simulink model "Quadcopter_CTC"  (R2021a)
settings: Solver=ode4  StartTime=0.0  StopTime=40  FixedStep=0.001  RelTol=1e-5
values from neighbouring files (symbols this model uses):
  IQ_x = 7.5e-3    (= 0.0075)    [Parameters.m]
  IQ_y = 7.5e-3    (= 0.0075)    [Parameters.m]
  IQ_z = 1.3e-2    (= 0.013)    [Parameters.m]
  mQ = 0.650    (= 0.65)    [Parameters.m]
libraries: pid_lib x4
settings Model: Creator=Mohamed Eid  LastModifiedBy=Mohamed Eid
settings DebuggingCC: SignalInfNanChecking=error

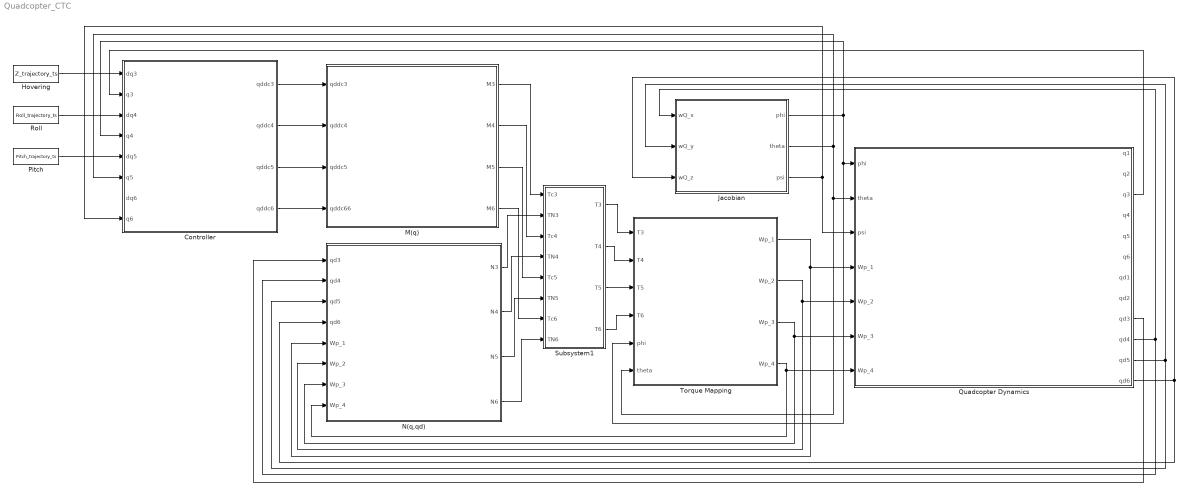
== system Quadcopter_CTC ==
  Controller : Subsystem
  Hovering : FromWorkspace  VariableName=Z_trajectory_ts  SampleTime=-1
  Jacobian : Subsystem
  M(q) : Subsystem
  N(q,qd) : Subsystem
      settings: MinAlgLoopOccurrences=on
  Pitch : FromWorkspace  VariableName=Pitch_trajectory_ts  SampleTime=-1
  Quadcopter Dynamics : Subsystem
      mask Display: image('C:\Users\Mohamed Eid\Desktop\Quadcopter Research\WhatsApp Image 2024-09-17 at 19.38.20.jpeg'); % Use "Edit Image" on toolstrip to change.
  Roll : FromWorkspace  VariableName=Roll_trajectory_ts  SampleTime=-1
  Subsystem1 : Subsystem
      settings: MinAlgLoopOccurrences=on
  Torque Mapping : Subsystem
      settings: MinAlgLoopOccurrences=on
  wires:
  Torque Mapping/3(Wp_3) -> N(q,qd)/7(Wp_3), Quadcopter Dynamics/6(Wp_3)
  Torque Mapping/2(Wp_2) -> N(q,qd)/6(Wp_2), Quadcopter Dynamics/5(Wp_2)
  Torque Mapping/1(Wp_1) -> N(q,qd)/5(Wp_1), Quadcopter Dynamics/4(Wp_1)
  Torque Mapping/4(Wp_4) -> N(q,qd)/8(Wp_4), Quadcopter Dynamics/7(Wp_4)
  Jacobian/1(phi) -> Torque Mapping/5(phi), Quadcopter Dynamics/1(phi), Controller/4(q4)
  Jacobian/2(theta) -> Torque Mapping/6(theta), Quadcopter Dynamics/2(theta), Controller/6(q5)
  Jacobian/3(psi) -> Quadcopter Dynamics/3(psi), Controller/8(q6)
  Quadcopter Dynamics/10(qd4) -> N(q,qd)/2(qd4), Jacobian/1(wQ_x)
  Quadcopter Dynamics/11(qd5) -> N(q,qd)/3(qd5), Jacobian/2(wQ_y)
  Quadcopter Dynamics/12(qd6) -> N(q,qd)/4(qd6), Jacobian/3(wQ_z)
  Controller/1(qddc3) -> M(q)/1(qddc3)
  Controller/2(qddc4) -> M(q)/2(qddc4)
  Controller/3(qddc5) -> M(q)/3(qddc5)
  Controller/4(qddc6) -> M(q)/4(qddc66)
  Quadcopter Dynamics/3(q3) -> Controller/2(q3)
  Quadcopter Dynamics/9(qd3) -> N(q,qd)/1(qd3)
  Subsystem1/1(T3) -> Torque Mapping/1(T3)
  Subsystem1/2(T4) -> Torque Mapping/2(T4)
  Subsystem1/3(T5) -> Torque Mapping/3(T5)
  Subsystem1/4(T6) -> Torque Mapping/4(T6)
  M(q)/1(M3) -> Subsystem1/1(Tc3)
  M(q)/2(M4) -> Subsystem1/3(Tc4)
  M(q)/3(M5) -> Subsystem1/5(Tc5)
  M(q)/4(M6) -> Subsystem1/7(Tc6)
  N(q,qd)/1(N3) -> Subsystem1/2(TN3)
  N(q,qd)/2(N4) -> Subsystem1/4(TN4)
  N(q,qd)/3(N5) -> Subsystem1/6(TN5)
  N(q,qd)/4(N6) -> Subsystem1/8(TN6)
  Hovering/1 -> Controller/1(dq3)
  Roll/1 -> Controller/3(dq4)
  Pitch/1 -> Controller/5(dq5)

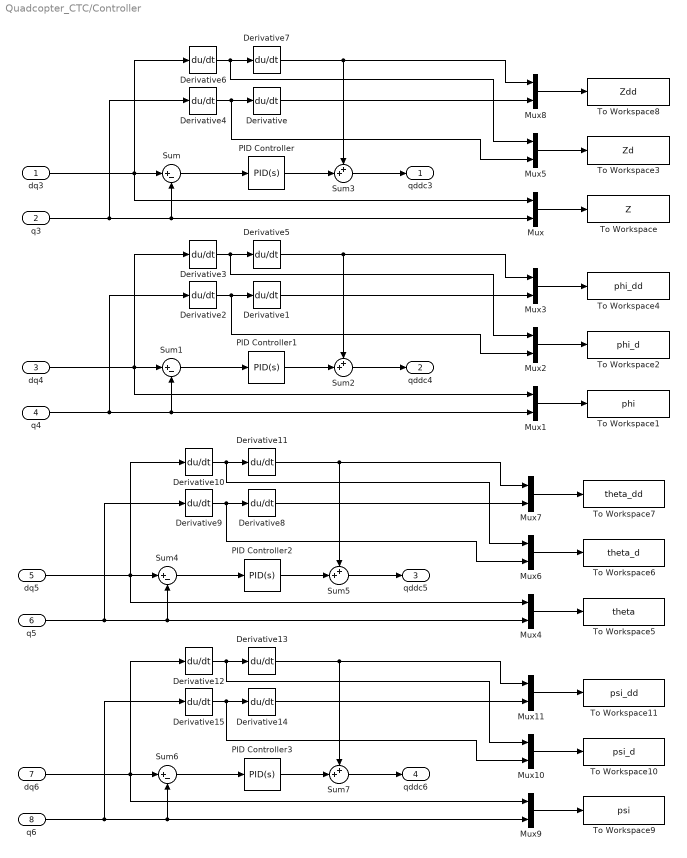
== system Quadcopter_CTC/Controller ==
  dq3 : Inport
  q3 : Inport  Port=2
  dq4 : Inport  Port=3
  q4 : Inport  Port=4
  dq5 : Inport  Port=5
  q5 : Inport  Port=6
  dq6 : Inport  Port=7
  q6 : Inport  Port=8
  Derivative{,1..15} (16 alike) : Derivative
  Mux{,1..11} (12 alike) : Mux  Inputs=2
  PID Controller : pid_lib/PID Controller  Controller=PID  Form=Parallel  TimeDomain=Continuous-time  UseExternalTs=off  SampleTime=-1  IntegratorMethod=Forward Euler  FilterMethod=Forward Euler  ControllerParametersSource=internal  P=2  I=0.6  D=20  UseFilter=on  N=3  TunerSelectOption=Transfer Function Based (PID Tuner App)  InitialConditionSource=internal  InitialConditionForIntegrator=0  InitialConditionForFilter=0  DifferentiatorICPrevScaledInput=0  ExternalReset=none  TrackingMode=off  Kt=1  LimitOutput=off  SatLimitsSource=internal  UpperSaturationLimit=inf  LowerSaturationLimit=-inf  LinearizeAsGain=on  AntiWindupMode=none  Kb=1  POutMin=[]  POutMax=[]  IOutMin=[]  IOutMax=[]  DOutMin=[]  DOutMax=[]  NOutMin=[]  NOutMax=[]  SumOutMin=[]  SumOutMax=[]  SaturationOutMin=[]  SaturationOutMax=[]  PParamMin=[]  PParamMax=[]  IParamMin=[]  IParamMax=[]  DParamMin=[]  DParamMax=[]  NParamMin=[]  NParamMax=[]  KbParamMin=[]  KbParamMax=[]  KtParamMin=[]  KtParamMax=[]  KbOutMin=[]  KbOutMax=[]  KtOutMin=[]  KtOutMax=[]  IntegratorOutMin=[]  IntegratorOutMax=[]  FilterOutMin=[]  FilterOutMax=[]  SumI1OutMin=[]  SumI1OutMax=[]  SumI2OutMin=[]  SumI2OutMax=[]  SumI3OutMin=[]  SumI3OutMax=[]  SumI4OutMin=[]  SumI4OutMax=[]  SumDOutMin=[]  SumDOutMax=[]  DifferentiatorOutMin=[]  DifferentiatorOutMax=[]  FilterDiffOutCoefMin=[]  FilterDiffOutCoefMax=[]  ReciprocalOutMin=[]  ReciprocalOutMax=[]  SumDenOutMin=[]  SumDenOutMax=[]  SumNumOutMin=[]  SumNumOutMax=[]  DivideOutMin=[]  DivideOutMax=[]  UdiffTsProdOutMin=[]  UdiffTsProdOutMax=[]  NTsProdOutMin=[]  NTsProdOutMax=[]  UintegralTsProdOutMin=[]  UintegralTsProdOutMax=[]  UngainTsProdOutMin=[]  UngainTsProdOutMax=[]  IntegratorContinuousStateAttributes=''  IntegratorStateMustResolveToSignalObject=off  IntegratorRTWStateStorageClass=Auto  FilterContinuousStateAttributes=''  FilterStateMustResolveToSignalObject=off  FilterRTWStateStorageClass=Auto  ParallelPVariant=InternalParameters  IdealPVariant=Disabled  IVariant=InternalParameters  DVariant=InternalParameters  IntegratorVariant=Continuous  SatVariant=Disabled  AWVariant=Passthrough  PCopyVariant=Disabled  TRVariant=Disabled  FdbkBlocksVariant=Forward  IdealPFdbkVariant=Disabled  SatFdbkVariant=Disabled  DerivativeFilterVariant=ContFilter  NVariant=InternalParameters  NCopyVariant=Disabled  FilterICVariant=InternalICsFilter  IntegratorICVariant=InternalICs  ExternalResetVariant=Disabled  TRSumVariant=Passthrough  SumFdbkVariant=Disabled  SumVariant=Sum_PID  TsampFilterVariant=InternalTs  TsampNgainVariant=Passthrough  TsampIntegralVariant=Passthrough  ExternalSaturationOutDataTypeStr=Inherit: Same as second input
  PID Controller1 : pid_lib/PID Controller  Controller=PID  Form=Parallel  TimeDomain=Continuous-time  UseExternalTs=off  SampleTime=-1  IntegratorMethod=Forward Euler  FilterMethod=Forward Euler  ControllerParametersSource=internal  P=2.62466504108734  I=0.153121092160732  D=9.99617214845314  UseFilter=on  N=1142.8279760416  TunerSelectOption=Transfer Function Based (PID Tuner App)  InitialConditionSource=internal  InitialConditionForIntegrator=0  InitialConditionForFilter=0  DifferentiatorICPrevScaledInput=0  ExternalReset=none  TrackingMode=off  Kt=1  LimitOutput=off  SatLimitsSource=internal  UpperSaturationLimit=inf  LowerSaturationLimit=-inf  LinearizeAsGain=on  AntiWindupMode=none  Kb=1  POutMin=[]  POutMax=[]  IOutMin=[]  IOutMax=[]  DOutMin=[]  DOutMax=[]  NOutMin=[]  NOutMax=[]  SumOutMin=[]  SumOutMax=[]  SaturationOutMin=[]  SaturationOutMax=[]  PParamMin=[]  PParamMax=[]  IParamMin=[]  IParamMax=[]  DParamMin=[]  DParamMax=[]  NParamMin=[]  NParamMax=[]  KbParamMin=[]  KbParamMax=[]  KtParamMin=[]  KtParamMax=[]  KbOutMin=[]  KbOutMax=[]  KtOutMin=[]  KtOutMax=[]  IntegratorOutMin=[]  IntegratorOutMax=[]  FilterOutMin=[]  FilterOutMax=[]  SumI1OutMin=[]  SumI1OutMax=[]  SumI2OutMin=[]  SumI2OutMax=[]  SumI3OutMin=[]  SumI3OutMax=[]  SumI4OutMin=[]  SumI4OutMax=[]  SumDOutMin=[]  SumDOutMax=[]  DifferentiatorOutMin=[]  DifferentiatorOutMax=[]  FilterDiffOutCoefMin=[]  FilterDiffOutCoefMax=[]  ReciprocalOutMin=[]  ReciprocalOutMax=[]  SumDenOutMin=[]  SumDenOutMax=[]  SumNumOutMin=[]  SumNumOutMax=[]  DivideOutMin=[]  DivideOutMax=[]  UdiffTsProdOutMin=[]  UdiffTsProdOutMax=[]  NTsProdOutMin=[]  NTsProdOutMax=[]  UintegralTsProdOutMin=[]  UintegralTsProdOutMax=[]  UngainTsProdOutMin=[]  UngainTsProdOutMax=[]  IntegratorContinuousStateAttributes=''  IntegratorStateMustResolveToSignalObject=off  IntegratorRTWStateStorageClass=Auto  FilterContinuousStateAttributes=''  FilterStateMustResolveToSignalObject=off  FilterRTWStateStorageClass=Auto  ParallelPVariant=InternalParameters  IdealPVariant=Disabled  IVariant=InternalParameters  DVariant=InternalParameters  IntegratorVariant=Continuous  SatVariant=Disabled  AWVariant=Passthrough  PCopyVariant=Disabled  TRVariant=Disabled  FdbkBlocksVariant=Forward  IdealPFdbkVariant=Disabled  SatFdbkVariant=Disabled  DerivativeFilterVariant=ContFilter  NVariant=InternalParameters  NCopyVariant=Disabled  FilterICVariant=InternalICsFilter  IntegratorICVariant=InternalICs  ExternalResetVariant=Disabled  TRSumVariant=Passthrough  SumFdbkVariant=Disabled  SumVariant=Sum_PID  TsampFilterVariant=InternalTs  TsampNgainVariant=Passthrough  TsampIntegralVariant=Passthrough  ExternalSaturationOutDataTypeStr=Inherit: Same as second input
  PID Controller2 : pid_lib/PID Controller  Controller=PID  Form=Parallel  TimeDomain=Continuous-time  UseExternalTs=off  SampleTime=-1  IntegratorMethod=Forward Euler  FilterMethod=Forward Euler  ControllerParametersSource=internal  P=2.39372296715018  I=0.133362896126307  D=9.54627029036672  UseFilter=on  N=1091.39224421761  TunerSelectOption=Transfer Function Based (PID Tuner App)  InitialConditionSource=internal  InitialConditionForIntegrator=0  InitialConditionForFilter=0  DifferentiatorICPrevScaledInput=0  ExternalReset=none  TrackingMode=off  Kt=1  LimitOutput=off  SatLimitsSource=internal  UpperSaturationLimit=inf  LowerSaturationLimit=-inf  LinearizeAsGain=on  AntiWindupMode=none  Kb=1  POutMin=[]  POutMax=[]  IOutMin=[]  IOutMax=[]  DOutMin=[]  DOutMax=[]  NOutMin=[]  NOutMax=[]  SumOutMin=[]  SumOutMax=[]  SaturationOutMin=[]  SaturationOutMax=[]  PParamMin=[]  PParamMax=[]  IParamMin=[]  IParamMax=[]  DParamMin=[]  DParamMax=[]  NParamMin=[]  NParamMax=[]  KbParamMin=[]  KbParamMax=[]  KtParamMin=[]  KtParamMax=[]  KbOutMin=[]  KbOutMax=[]  KtOutMin=[]  KtOutMax=[]  IntegratorOutMin=[]  IntegratorOutMax=[]  FilterOutMin=[]  FilterOutMax=[]  SumI1OutMin=[]  SumI1OutMax=[]  SumI2OutMin=[]  SumI2OutMax=[]  SumI3OutMin=[]  SumI3OutMax=[]  SumI4OutMin=[]  SumI4OutMax=[]  SumDOutMin=[]  SumDOutMax=[]  DifferentiatorOutMin=[]  DifferentiatorOutMax=[]  FilterDiffOutCoefMin=[]  FilterDiffOutCoefMax=[]  ReciprocalOutMin=[]  ReciprocalOutMax=[]  SumDenOutMin=[]  SumDenOutMax=[]  SumNumOutMin=[]  SumNumOutMax=[]  DivideOutMin=[]  DivideOutMax=[]  UdiffTsProdOutMin=[]  UdiffTsProdOutMax=[]  NTsProdOutMin=[]  NTsProdOutMax=[]  UintegralTsProdOutMin=[]  UintegralTsProdOutMax=[]  UngainTsProdOutMin=[]  UngainTsProdOutMax=[]  IntegratorContinuousStateAttributes=''  IntegratorStateMustResolveToSignalObject=off  IntegratorRTWStateStorageClass=Auto  FilterContinuousStateAttributes=''  FilterStateMustResolveToSignalObject=off  FilterRTWStateStorageClass=Auto  ParallelPVariant=InternalParameters  IdealPVariant=Disabled  IVariant=InternalParameters  DVariant=InternalParameters  IntegratorVariant=Continuous  SatVariant=Disabled  AWVariant=Passthrough  PCopyVariant=Disabled  TRVariant=Disabled  FdbkBlocksVariant=Forward  IdealPFdbkVariant=Disabled  SatFdbkVariant=Disabled  DerivativeFilterVariant=ContFilter  NVariant=InternalParameters  NCopyVariant=Disabled  FilterICVariant=InternalICsFilter  IntegratorICVariant=InternalICs  ExternalResetVariant=Disabled  TRSumVariant=Passthrough  SumFdbkVariant=Disabled  SumVariant=Sum_PID  TsampFilterVariant=InternalTs  TsampNgainVariant=Passthrough  TsampIntegralVariant=Passthrough  ExternalSaturationOutDataTypeStr=Inherit: Same as second input
  PID Controller3 : pid_lib/PID Controller  Controller=PID  Form=Parallel  TimeDomain=Continuous-time  UseExternalTs=off  SampleTime=-1  IntegratorMethod=Forward Euler  FilterMethod=Forward Euler  ControllerParametersSource=internal  P=2.62466504110809  I=0.153121092161943  D=9.99617214853218  UseFilter=on  N=1142.8279760416  TunerSelectOption=Transfer Function Based (PID Tuner App)  InitialConditionSource=internal  InitialConditionForIntegrator=0  InitialConditionForFilter=0  DifferentiatorICPrevScaledInput=0  ExternalReset=none  TrackingMode=off  Kt=1  LimitOutput=off  SatLimitsSource=internal  UpperSaturationLimit=inf  LowerSaturationLimit=-inf  LinearizeAsGain=on  AntiWindupMode=none  Kb=1  POutMin=[]  POutMax=[]  IOutMin=[]  IOutMax=[]  DOutMin=[]  DOutMax=[]  NOutMin=[]  NOutMax=[]  SumOutMin=[]  SumOutMax=[]  SaturationOutMin=[]  SaturationOutMax=[]  PParamMin=[]  PParamMax=[]  IParamMin=[]  IParamMax=[]  DParamMin=[]  DParamMax=[]  NParamMin=[]  NParamMax=[]  KbParamMin=[]  KbParamMax=[]  KtParamMin=[]  KtParamMax=[]  KbOutMin=[]  KbOutMax=[]  KtOutMin=[]  KtOutMax=[]  IntegratorOutMin=[]  IntegratorOutMax=[]  FilterOutMin=[]  FilterOutMax=[]  SumI1OutMin=[]  SumI1OutMax=[]  SumI2OutMin=[]  SumI2OutMax=[]  SumI3OutMin=[]  SumI3OutMax=[]  SumI4OutMin=[]  SumI4OutMax=[]  SumDOutMin=[]  SumDOutMax=[]  DifferentiatorOutMin=[]  DifferentiatorOutMax=[]  FilterDiffOutCoefMin=[]  FilterDiffOutCoefMax=[]  ReciprocalOutMin=[]  ReciprocalOutMax=[]  SumDenOutMin=[]  SumDenOutMax=[]  SumNumOutMin=[]  SumNumOutMax=[]  DivideOutMin=[]  DivideOutMax=[]  UdiffTsProdOutMin=[]  UdiffTsProdOutMax=[]  NTsProdOutMin=[]  NTsProdOutMax=[]  UintegralTsProdOutMin=[]  UintegralTsProdOutMax=[]  UngainTsProdOutMin=[]  UngainTsProdOutMax=[]  IntegratorContinuousStateAttributes=''  IntegratorStateMustResolveToSignalObject=off  IntegratorRTWStateStorageClass=Auto  FilterContinuousStateAttributes=''  FilterStateMustResolveToSignalObject=off  FilterRTWStateStorageClass=Auto  ParallelPVariant=InternalParameters  IdealPVariant=Disabled  IVariant=InternalParameters  DVariant=InternalParameters  IntegratorVariant=Continuous  SatVariant=Disabled  AWVariant=Passthrough  PCopyVariant=Disabled  TRVariant=Disabled  FdbkBlocksVariant=Forward  IdealPFdbkVariant=Disabled  SatFdbkVariant=Disabled  DerivativeFilterVariant=ContFilter  NVariant=InternalParameters  NCopyVariant=Disabled  FilterICVariant=InternalICsFilter  IntegratorICVariant=InternalICs  ExternalResetVariant=Disabled  TRSumVariant=Passthrough  SumFdbkVariant=Disabled  SumVariant=Sum_PID  TsampFilterVariant=InternalTs  TsampNgainVariant=Passthrough  TsampIntegralVariant=Passthrough  ExternalSaturationOutDataTypeStr=Inherit: Same as second input
  Sum{,1,4,6} (4 alike) : Sum  Inputs=|+-
  Sum{2..3,5,7} (4 alike) : Sum  Inputs=++|
  To Workspace : ToWorkspace  VariableName=Z  SaveFormat=Timeseries  SampleTime=-1
  To Workspace1 : ToWorkspace  VariableName=phi  SaveFormat=Timeseries  SampleTime=-1
  To Workspace10 : ToWorkspace  VariableName=psi_d  SaveFormat=Timeseries  SampleTime=-1
  To Workspace11 : ToWorkspace  VariableName=psi_dd  SaveFormat=Timeseries  SampleTime=-1
  To Workspace2 : ToWorkspace  VariableName=phi_d  SaveFormat=Timeseries  SampleTime=-1
  To Workspace3 : ToWorkspace  VariableName=Zd  SaveFormat=Timeseries  SampleTime=-1
  To Workspace4 : ToWorkspace  VariableName=phi_dd  SaveFormat=Timeseries  SampleTime=-1
  To Workspace5 : ToWorkspace  VariableName=theta  SaveFormat=Timeseries  SampleTime=-1
  To Workspace6 : ToWorkspace  VariableName=theta_d  SaveFormat=Timeseries  SampleTime=-1
  To Workspace7 : ToWorkspace  VariableName=theta_dd  SaveFormat=Timeseries  SampleTime=-1
  To Workspace8 : ToWorkspace  VariableName=Zdd  SaveFormat=Timeseries  SampleTime=-1
  To Workspace9 : ToWorkspace  VariableName=psi  SaveFormat=Timeseries  SampleTime=-1
  qddc3 : Outport
  qddc4 : Outport  Port=2
  qddc5 : Outport  Port=3
  qddc6 : Outport  Port=4
  wires:
  Derivative6/1 -> Mux5/1, Derivative7/1
  q3/1 -> Derivative4/1, Sum/2, Mux/2
  Derivative7/1 -> Sum3/1, Mux8/1
  Mux8/1 -> To Workspace8/1
  Mux/1 -> To Workspace/1
  Mux5/1 -> To Workspace3/1
  Sum3/1 -> qddc3/1
  Derivative/1 -> Mux8/2
  dq3/1 -> Derivative6/1, Mux/1, Sum/1
  Derivative4/1 -> Mux5/2, Derivative/1
  Derivative2/1 -> Derivative1/1, Mux2/2
  dq4/1 -> Sum1/1, Mux1/1, Derivative3/1
  Derivative1/1 -> Mux3/2
  Sum2/1 -> qddc4/1
  Mux2/1 -> To Workspace2/1
  Mux1/1 -> To Workspace1/1
  Mux3/1 -> To Workspace4/1
  Derivative5/1 -> Mux3/1, Sum2/1
  q4/1 -> Mux1/2, Sum1/2, Derivative2/1
  Derivative3/1 -> Derivative5/1, Mux2/1
  Derivative10/1 -> Mux6/1, Derivative11/1
  q5/1 -> Derivative9/1, Sum4/2, Mux4/2
  Derivative11/1 -> Sum5/1, Mux7/1
  Mux7/1 -> To Workspace7/1
  PID Controller2/1 -> Sum5/2
  Mux4/1 -> To Workspace5/1
  Mux6/1 -> To Workspace6/1
  Sum5/1 -> qddc5/1
  Derivative8/1 -> Mux7/2
  dq5/1 -> Derivative10/1, Mux4/1, Sum4/1
  Derivative9/1 -> Mux6/2, Derivative8/1
  Sum4/1 -> PID Controller2/1
  Sum6/1 -> PID Controller3/1
  Derivative15/1 -> Derivative14/1, Mux10/2
  dq6/1 -> Sum6/1, Mux9/1, Derivative12/1
  Derivative14/1 -> Mux11/2
  Sum7/1 -> qddc6/1
  Mux10/1 -> To Workspace10/1
  Mux9/1 -> To Workspace9/1
  PID Controller3/1 -> Sum7/2
  Mux11/1 -> To Workspace11/1
  Derivative13/1 -> Mux11/1, Sum7/1
  q6/1 -> Mux9/2, Sum6/2, Derivative15/1
  Derivative12/1 -> Derivative13/1, Mux10/1
  PID Controller1/1 -> Sum2/2
  Sum1/1 -> PID Controller1/1
  PID Controller/1 -> Sum3/2
  Sum/1 -> PID Controller/1

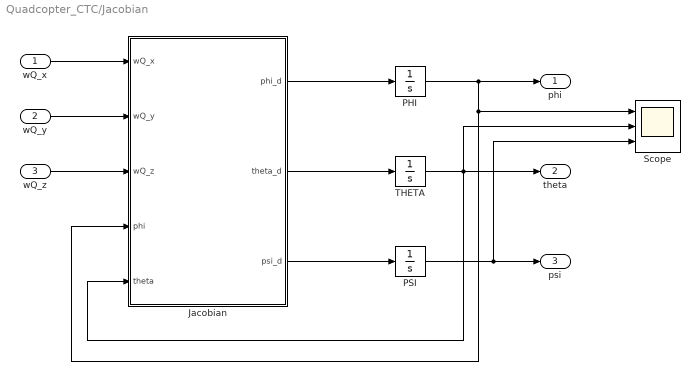
== system Quadcopter_CTC/Jacobian ==
  wQ_x : Inport
  wQ_y : Inport  Port=2
  wQ_z : Inport  Port=3
  Jacobian : MATLAB Function  TreatAsAtomicUnit=on
  PHI : Integrator
  PSI : Integrator
  Scope : Scope  NumInputPorts=3
  THETA : Integrator
  phi : Outport
  theta : Outport  Port=2
  psi : Outport  Port=3
  wires:
  wQ_x/1 -> Jacobian/1(wQ_x)
  wQ_y/1 -> Jacobian/2(wQ_y)
  wQ_z/1 -> Jacobian/3(wQ_z)
  Jacobian/1(phi_d) -> PHI/1
  PHI/1 -> Scope/1, Jacobian/4(phi), phi/1
  Jacobian/2(theta_d) -> THETA/1
  THETA/1 -> Scope/2, theta/1, Jacobian/5(theta)
  Jacobian/3(psi_d) -> PSI/1
  PSI/1 -> Scope/3, psi/1

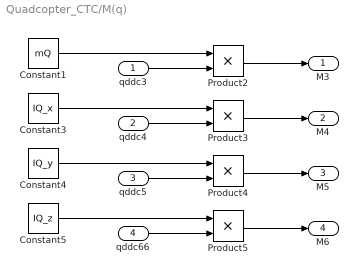
== system Quadcopter_CTC/M(q) ==
  qddc3 : Inport
  qddc4 : Inport  Port=2
  qddc5 : Inport  Port=3
  qddc66 : Inport  Port=4
  Constant1 : Constant  Value=mQ
  Constant3 : Constant  Value=IQ_x
  Constant4 : Constant  Value=IQ_y
  Constant5 : Constant  Value=IQ_z
  Product{2..5} (4 alike) : Product
  M3 : Outport
  M4 : Outport  Port=2
  M5 : Outport  Port=3
  M6 : Outport  Port=4
  wires:
  Constant5/1 -> Product5/1
  Constant4/1 -> Product4/1
  Constant3/1 -> Product3/1
  qddc3/1 -> Product2/2
  qddc4/1 -> Product3/2
  qddc5/1 -> Product4/2
  qddc66/1 -> Product5/2
  Product2/1 -> M3/1
  Product3/1 -> M4/1
  Product4/1 -> M5/1
  Product5/1 -> M6/1
  Constant1/1 -> Product2/1

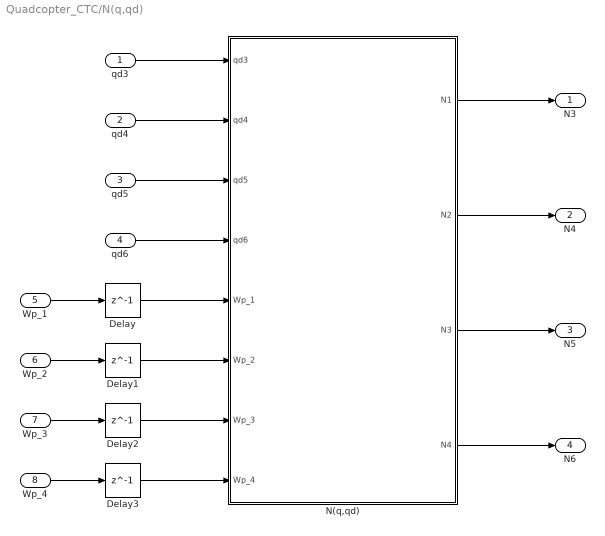
== system Quadcopter_CTC/N(q,qd) ==
  qd3 : Inport
  qd4 : Inport  Port=2
  qd5 : Inport  Port=3
  qd6 : Inport  Port=4
  Wp_1 : Inport  Port=5
  Wp_2 : Inport  Port=6
  Wp_3 : Inport  Port=7
  Wp_4 : Inport  Port=8
  Delay{,1..3} (4 alike) : Delay  DelayLength=1  InitialCondition=0
  N(q,qd) : MATLAB Function  TreatAsAtomicUnit=on
  N3 : Outport
  N4 : Outport  Port=2
  N5 : Outport  Port=3
  N6 : Outport  Port=4
  wires:
  qd6/1 -> N(q,qd)/4(qd6)
  qd5/1 -> N(q,qd)/3(qd5)
  qd4/1 -> N(q,qd)/2(qd4)
  qd3/1 -> N(q,qd)/1(qd3)
  Wp_1/1 -> Delay/1
  Wp_4/1 -> Delay3/1
  Wp_3/1 -> Delay2/1
  Wp_2/1 -> Delay1/1
  N(q,qd)/1(N1) -> N3/1
  N(q,qd)/2(N2) -> N4/1
  N(q,qd)/3(N3) -> N5/1
  N(q,qd)/4(N4) -> N6/1
  Delay/1 -> N(q,qd)/5(Wp_1)
  Delay1/1 -> N(q,qd)/6(Wp_2)
  Delay2/1 -> N(q,qd)/7(Wp_3)
  Delay3/1 -> N(q,qd)/8(Wp_4)

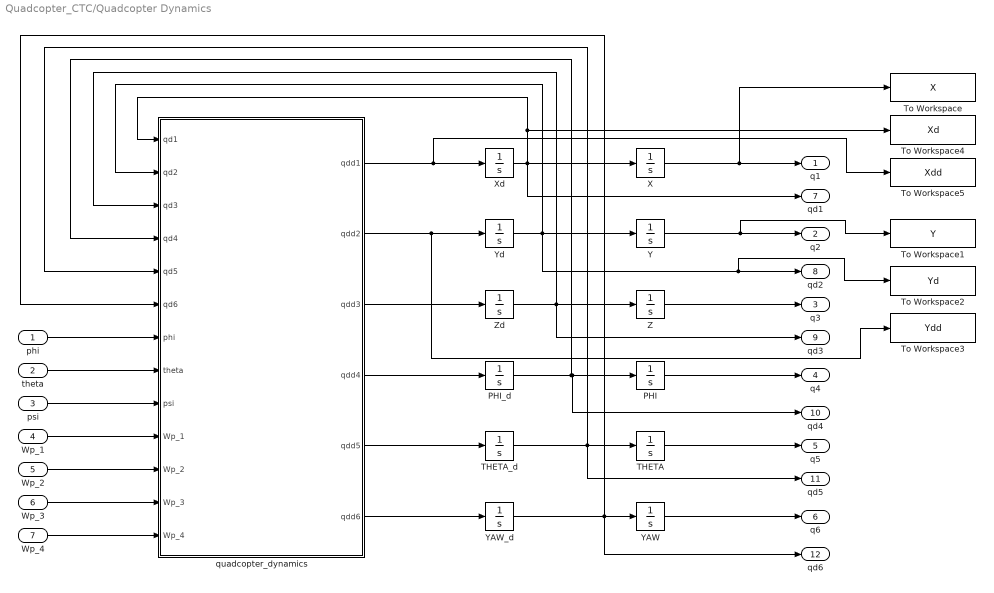
== system Quadcopter_CTC/Quadcopter Dynamics ==
  phi : Inport
  theta : Inport  Port=2
  psi : Inport  Port=3
  Wp_1 : Inport  Port=4
  Wp_2 : Inport  Port=5
  Wp_3 : Inport  Port=6
  Wp_4 : Inport  Port=7
  PHI : Integrator  UpperSaturationLimit=pi/2  LowerSaturationLimit=-pi/2  WrapState=on
  PHI_d : Integrator
  THETA : Integrator  WrapState=on
  THETA_d : Integrator
  To Workspace : ToWorkspace  VariableName=X  SaveFormat=Timeseries  SampleTime=-1
  To Workspace1 : ToWorkspace  VariableName=Y  SaveFormat=Timeseries  SampleTime=-1
  To Workspace2 : ToWorkspace  VariableName=Yd  SaveFormat=Timeseries  SampleTime=-1
  To Workspace3 : ToWorkspace  VariableName=Ydd  SaveFormat=Timeseries  SampleTime=-1
  To Workspace4 : ToWorkspace  VariableName=Xd  SaveFormat=Timeseries  SampleTime=-1
  To Workspace5 : ToWorkspace  VariableName=Xdd  SaveFormat=Timeseries  SampleTime=-1
  X : Integrator
  Xd : Integrator
  Y : Integrator
  YAW : Integrator  WrapState=on
  YAW_d : Integrator
  Yd : Integrator
  Z : Integrator  LimitOutput=on  LowerSaturationLimit=0
  Zd : Integrator
  quadcopter_dynamics : MATLAB Function  TreatAsAtomicUnit=on
  q1 : Outport
  q2 : Outport  Port=2
  q3 : Outport  Port=3
  q4 : Outport  Port=4
  q5 : Outport  Port=5
  q6 : Outport  Port=6
  qd1 : Outport  Port=7
  qd2 : Outport  Port=8
  qd3 : Outport  Port=9
  qd4 : Outport  Port=10
  qd5 : Outport  Port=11
  qd6 : Outport  Port=12
  wires:
  theta/1 -> quadcopter_dynamics/8(theta)
  phi/1 -> quadcopter_dynamics/7(phi)
  psi/1 -> quadcopter_dynamics/9(psi)
  Wp_4/1 -> quadcopter_dynamics/13(Wp_4)
  Wp_3/1 -> quadcopter_dynamics/12(Wp_3)
  Wp_2/1 -> quadcopter_dynamics/11(Wp_2)
  Wp_1/1 -> quadcopter_dynamics/10(Wp_1)
  quadcopter_dynamics/1(qdd1) -> To Workspace5/1, Xd/1
  Xd/1 -> qd1/1, quadcopter_dynamics/1(qd1), To Workspace4/1, X/1
  X/1 -> To Workspace/1, q1/1
  Y/1 -> To Workspace1/1, q2/1
  Yd/1 -> To Workspace2/1, qd2/1, Y/1, quadcopter_dynamics/2(qd2)
  quadcopter_dynamics/2(qdd2) -> To Workspace3/1, Yd/1
  quadcopter_dynamics/3(qdd3) -> Zd/1
  Zd/1 -> qd3/1, Z/1, quadcopter_dynamics/3(qd3)
  Z/1 -> q3/1
  PHI/1 -> q4/1
  quadcopter_dynamics/4(qdd4) -> PHI_d/1
  quadcopter_dynamics/5(qdd5) -> THETA_d/1
  THETA_d/1 -> qd5/1, THETA/1, quadcopter_dynamics/5(qd5)
  THETA/1 -> q5/1
  YAW/1 -> q6/1
  YAW_d/1 -> qd6/1, quadcopter_dynamics/6(qd6), YAW/1
  quadcopter_dynamics/6(qdd6) -> YAW_d/1
  PHI_d/1 -> quadcopter_dynamics/4(qd4), qd4/1, PHI/1

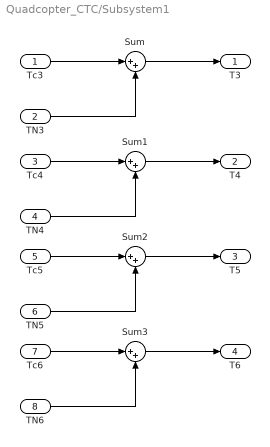
== system Quadcopter_CTC/Subsystem1 ==
  Tc3 : Inport
  TN3 : Inport  Port=2
  Tc4 : Inport  Port=3
  TN4 : Inport  Port=4
  Tc5 : Inport  Port=5
  TN5 : Inport  Port=6
  Tc6 : Inport  Port=7
  TN6 : Inport  Port=8
  Sum{,1..3} (4 alike) : Sum  Inputs=|++
  T3 : Outport
  T4 : Outport  Port=2
  T5 : Outport  Port=3
  T6 : Outport  Port=4
  wires:
  Sum/1 -> T3/1
  Tc3/1 -> Sum/1
  TN3/1 -> Sum/2
  TN4/1 -> Sum1/2
  Tc4/1 -> Sum1/1
  Sum1/1 -> T4/1
  Sum2/1 -> T5/1
  Tc5/1 -> Sum2/1
  TN5/1 -> Sum2/2
  TN6/1 -> Sum3/2
  Tc6/1 -> Sum3/1
  Sum3/1 -> T6/1

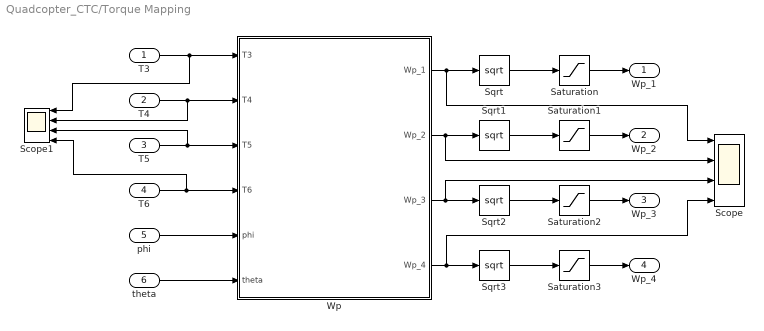
== system Quadcopter_CTC/Torque Mapping ==
  T3 : Inport
  T4 : Inport  Port=2
  T5 : Inport  Port=3
  T6 : Inport  Port=4
  phi : Inport  Port=5
  theta : Inport  Port=6
  Saturation{,1..3} (4 alike) : Saturate  UpperLimit=500  LowerLimit=0
  Scope : Scope  NumInputPorts=4
  Scope1 : Scope  NumInputPorts=4
  Sqrt{,1..3} (4 alike) : Sqrt  OutputSignalType=real  SaturateOnIntegerOverflow=on
  Wp : MATLAB Function  TreatAsAtomicUnit=on
  Wp_1 : Outport
  Wp_2 : Outport  Port=2
  Wp_3 : Outport  Port=3
  Wp_4 : Outport  Port=4
  wires:
  phi/1 -> Wp/5(phi)
  theta/1 -> Wp/6(theta)
  Wp/1(Wp_1) -> Scope/1, Sqrt/1
  Wp/2(Wp_2) -> Sqrt1/1, Scope/2
  Wp/3(Wp_3) -> Sqrt2/1, Scope/3
  Wp/4(Wp_4) -> Sqrt3/1, Scope/4
  T3/1 -> Scope1/1, Wp/1(T3)
  T4/1 -> Scope1/2, Wp/2(T4)
  T5/1 -> Scope1/3, Wp/3(T5)
  T6/1 -> Scope1/4, Wp/4(T6)
  Sqrt/1 -> Saturation/1
  Sqrt1/1 -> Saturation1/1
  Sqrt2/1 -> Saturation2/1
  Sqrt3/1 -> Saturation3/1
  Saturation/1 -> Wp_1/1
  Saturation1/1 -> Wp_2/1
  Saturation2/1 -> Wp_3/1
  Saturation3/1 -> Wp_4/1

== matlab function Quadcopter_CTC/N(q,qd)/N(q,qd) ==
  data: N1 output; qd3 input; qd4 input; qd5 input; qd6 input; Wp_1 input; Wp_2 input; Wp_3 input; Wp_4 input; N2 output; N3 output; N4 output
function [N1,N2,N3,N4] = non_linearity_matrix(qd3,qd4,qd5,qd6,Wp_1,Wp_2,Wp_3,Wp_4)

%Output
N1 = (3*qd3)/20 + 12753/2000;
N2 = qd4^2/10 + (3*qd5*qd6)/400 - qd5*((3*Wp_1)/50000 - (3*Wp_2)/50000 + (3*Wp_3)/50000 - (3*Wp_4)/50000 + (13*qd6)/1000);
N3 = qd5^2/10 - (3*qd4*qd6)/400 + qd4*((3*Wp_1)/50000 - (3*Wp_2)/50000 + (3*Wp_3)/50000 - (3*Wp_4)/50000 + (13*qd6)/1000);
N4 = (3*qd6^2)/20;

end

== matlab function Quadcopter_CTC/Quadcopter Dynamics/quadcopter_dynamics ==
  data: qdd1 output; qd1 input; qd2 input; qd3 input; qd4 input; qd5 input; qd6 input; phi input; theta input; psi input; Wp_1 input; Wp_2 input; Wp_3 input; Wp_4 input; qdd2 output; qdd3 output; qdd4 output; qdd5 output; qdd6 output
function [qdd1,qdd2,qdd3,qdd4,qdd5,qdd6] = quadcopter_dynamics(qd1,qd2,qd3,qd4,qd5,qd6,phi,theta,psi,Wp_1,Wp_2,Wp_3,Wp_4)

%Output
qdd1 = (2886915447535545*Wp_1^2*sin(phi)*sin(psi))/59951918239556042752 - (2*qd1)/13 + (2886915447535545*Wp_2^2*sin(phi)*sin(psi))/59951918239556042752 + (2886915447535545*Wp_3^2*sin(phi)*sin(psi))/59951918239556042752 + (2886915447535545*Wp_4^2*sin(phi)*sin(psi))/59951918239556042752 + (2886915447535545*Wp_1^2*cos(phi)*cos(psi)*sin(theta))/59951918239556042752 + (2886915447535545*Wp_2^2*cos(phi)*cos(psi)*sin(theta))/59951918239556042752 + (2886915447535545*Wp_3^2*cos(phi)*cos(psi)*sin(theta))/59951918239556042752 + (2886915447535545*Wp_4^2*cos(phi)*cos(psi)*sin(theta))/59951918239556042752;
qdd2 = (2886915447535545*Wp_1^2*cos(phi)*sin(psi)*sin(theta))/59951918239556042752 - (2886915447535545*Wp_1^2*cos(psi)*sin(phi))/59951918239556042752 - (2886915447535545*Wp_2^2*cos(psi)*sin(phi))/59951918239556042752 - (2886915447535545*Wp_3^2*cos(psi)*sin(phi))/59951918239556042752 - (2886915447535545*Wp_4^2*cos(psi)*sin(phi))/59951918239556042752 - (2*qd2)/13 + (2886915447535545*Wp_2^2*cos(phi)*sin(psi)*sin(theta))/59951918239556042752 + (2886915447535545*Wp_3^2*cos(phi)*sin(psi)*sin(theta))/59951918239556042752 + (2886915447535545*Wp_4^2*cos(phi)*sin(psi)*sin(theta))/59951918239556042752;
qdd3 = (2886915447535545*cos(phi)*cos(theta)*Wp_1^2)/59951918239556042752 + (2886915447535545*cos(phi)*cos(theta)*Wp_2^2)/59951918239556042752 + (2886915447535545*cos(phi)*cos(theta)*Wp_3^2)/59951918239556042752 + (2886915447535545*cos(phi)*cos(theta)*Wp_4^2)/59951918239556042752 - (3*qd3)/13 - 981/100;
qdd4 = (212476976938616125*Wp_2^2)/221360928884514619392 - (qd5*Wp_2)/125 + (Wp_1*qd5)/125 + (Wp_3*qd5)/125 - (Wp_4*qd5)/125 + (11*qd5*qd6)/15 - (212476976938616125*Wp_4^2)/221360928884514619392 - (40*qd4^2)/3;
qdd5 = (212476976938616125*Wp_3^2)/221360928884514619392 - (qd4*Wp_3)/125 - (Wp_1*qd4)/125 + (Wp_2*qd4)/125 + (Wp_4*qd4)/125 - (11*qd4*qd6)/15 - (212476976938616125*Wp_1^2)/221360928884514619392 - (40*qd5^2)/3;
qdd6 = (221360928884514625*Wp_1^2)/3836922767331586736128 + (221360928884514625*Wp_3^2)/3836922767331586736128 - (221360928884514625*Wp_2^2)/3836922767331586736128 - (221360928884514625*Wp_4^2)/3836922767331586736128 - (150*qd6^2)/13;

end

== matlab function Quadcopter_CTC/Torque Mapping/Wp ==
  data: T3 input; T4 input; T5 input; T6 input; phi input; Wp_1 output; theta input; Wp_2 output; Wp_3 output; Wp_4 output
function [Wp_1,Wp_2,Wp_3,Wp_4] = torque_mapping(T3,T4,T5,T6,phi,theta)

%Output
Wp_1 = (4611686018427387904*(15050912314145810574002460743465*T3 - 130877498383876605679486926816384*T5*cos(phi)*cos(theta) + 628124740577018516152703024807040*T6*cos(phi)*cos(theta)))/(8690142251842099598340571732034872128542792685*cos(phi)*cos(theta));
Wp_2 = (4611686018427387904*(15050912314145810574002460743465*T3 + 130877498383876605679486926816384*T4*cos(phi)*cos(theta) - 628124740577018516152703024807040*T6*cos(phi)*cos(theta)))/(8690142251842099598340571732034872128542792685*cos(phi)*cos(theta));
Wp_3 = (4611686018427387904*(15050912314145810574002460743465*T3 + 130877498383876605679486926816384*T5*cos(phi)*cos(theta) + 628124740577018516152703024807040*T6*cos(phi)*cos(theta)))/(8690142251842099598340571732034872128542792685*cos(phi)*cos(theta));
Wp_4 = -(4611686018427387904*(130877498383876605679486926816384*T4*cos(phi)*cos(theta) - 15050912314145810574002460743465*T3 + 628124740577018516152703024807040*T6*cos(phi)*cos(theta)))/(8690142251842099598340571732034872128542792685*cos(phi)*cos(theta));

end

== matlab function Quadcopter_CTC/Jacobian/Jacobian ==
  data: wQ_x input; phi_d output; wQ_y input; wQ_z input; phi input; theta input; theta_d output; psi_d output
function [phi_d,theta_d,psi_d] = jacobian_matrix(wQ_x,wQ_y,wQ_z,phi,theta)

%Output
phi_d = wQ_x + sin(phi)*tan(theta)*wQ_y + cos(phi)*tan(theta)*wQ_z;
theta_d = cos(phi)*wQ_y - sin(phi)*wQ_z;
psi_d = (sin(phi)/cos(theta))*wQ_y + (cos(phi)/cos(theta))*wQ_z;

end
